simulink model "HvCoorn"  (R2022b)
settings: configuration reference "Icar05FusaMdlCfg" (kept outside this file)
undefined symbols (not defined in the file): BMSActSt_ACChrg, BMSActSt_DCChrg, BMSActSt_disconnect, BMSActSt_offline, BMSActSt_online, BMSActSt_undefined, BMSMainNegRlySt_Clsd_SC, BMSMainNegRlySt_Open_SC, BMSMainNegRlySt_StuckInClsd_SC, BMSMainNegRlySt_StuckInOpen_SC, BMSMainPosRlySt_Clsd_SC, BMSMainPosRlySt_Open_SC, BMSMainPosRlySt_StuckInClsd_SC, BMSPrecRlySt_StuckInOpen_SC, BMSReqSt_ACChrg, BMSReqSt_DCChrg, BMSReqSt_emergencyOffline, BMSReqSt_offline, BMSReqSt_online, Chrg_stCycleBookMod_SC, Chrg_stSingleBookMod_SC, CmpgMod_stInactv_SC, DCDCActSt_buck, DCDCActSt_connected, DCDCActSt_disconnected, DCDCReqSt_buck, DCDCReqSt_standby, EngStrtStop_RefuModDft_SC, EPBActSt_Appld_SC, GearLvr_stDrvGearD_SC, GearLvr_stDrvGearN_SC, GearLvr_stDrvGearP_SC, GearLvr_stDrvGearR_SC, hpp_bACChargeLinkIni_C, hpp_bACChargeLinkOKIni_C, hpp_bAcChgEnaIni_C, hpp_bAcChgPauseIni_C, hpp_bAcLinkTempErrIni_C, hpp_bBattWarmReqIni_C, hpp_bHvilHwErrIni_C, hpp_bHvilStOkIni_C, hpp_bHvRelayClsActIni_C, hpp_bHvRelayOpnActIni_C, hpp_bHvRelayStuckIni_C, hpp_bParked4ChDchgIni_C, hpp_bRemLvBatMntnReqIni_C, hpp_bStartUpReqIni_C, hpp_stHvilCanIni_C, hpp_stWarmTimeCfgRespIni_C, HvCoorn_bAuthEnaSwt_C, HvCoorn_bAuthFailSpdLimOvrd_C, HvCoorn_bAuthFailSpdLimOvrdVal_C, HvCoorn_bAuthStrt_C, HvCoorn_bBMSUnexpdDcnctFailEna_C, HvCoorn_bBuck2RdyBypDCDCEna_C, HvCoorn_bDCChrgFctCfg_C, HvCoorn_bDcChrgWkupEnaChrgLink_C, HvCoorn_bDCDcnct4ACEna_C, HvCoorn_bDCNotBuck2ShtdwnEna_C, HvCoorn_bDrvrLevNotRdyEna_C ... (+295)
libraries: ITKLib x213, simulink x61
(part 5 of 12)

== system HvCoorn/HvCoorn/HVP_HighVoltagePowerOnOffProcedure/A04_HVReq2DCBuckCal ==
  note: Documentation
  icfm_uAct : Inport
  icdc_uHvAct : Inport  Port=2
  icfm_stMode : Inport  Port=3
  icdc_stMode : Inport  Port=4
  icobc_stOBCMode : Inport  Port=5
  HvCoorn_stHVPOld : Inport  Port=6
  icobc_stChrgrCnct : Inport  Port=7
  idi_bKeyOn : Inport  Port=8
  HvCoorn_bStartUpReq : Inport  Port=9
  HvCoorn_bHvRlyClsAct : Inport  Port=10
  icrm_uAct : Inport  Port=11
  icrm_stMode : Inport  Port=12
  icbms_stDcChrg : Inport  Port=13
  icbms_stDcChrgrCnct : Inport  Port=14
  HvCoorn_stStartUpReq : Inport  Port=15
  icisg_uAct : Inport  Port=16
  VehCfg_bFrntMotByp : Inport  Port=17
  AND : Logic  OutDataTypeStr=boolean
  Constant1 : Constant  Description=[2]  Value=OBCChrgrCnctnSt_PtlCnct_SC
      settings: AttributesFormatString=%<Description>
  Constant10 : Constant  Description=[1]  Value=OBCChrgrCnctnSt_Cnct_SC
      settings: AttributesFormatString=%<Description>
  Copyright : simulink/Model-Wide Utilities/Model Info  Frame=on  DisplayStringWithTags=|  HorizontalTextAlignment=Left  LeftAlignmentValue=0.02
      | © ITK Engineering Technology (Wu Xi) Co., Ltd. (ITKC)
      | 
      | Model Version: %<ModelVersion>
      | Date: %<LastModificationDate>
  Equal : RelationalOperator  Operator=>  OutDataTypeStr=boolean  RndMeth=Simplest  InputSameDT=off
  InlineDescription : ITKLib/Special/InlineDescription  Tag=HideFromReport  Description=高压请求跳转至DCDC Buck  ShowInLibBrowser=0  RefreshPar=0
      settings: SourceProductName=ITKC_Lib
  Logical Operator1 : Logic  Inputs=3  AllPortsSameDT=off  OutDataTypeStr=boolean
  Logical Operator{5..7,10} (4 alike) : Logic  Operator=NOT  Inputs=1  AllPortsSameDT=off  OutDataTypeStr=boolean
  Logical Operator12 : Logic  Inputs=5  AllPortsSameDT=off  OutDataTypeStr=boolean
  Logical Operator{2..3,9,13,16..18} (7 alike) : Logic  Operator=OR  AllPortsSameDT=off  OutDataTypeStr=boolean
  Logical Operator{4,8,15,20} (4 alike) : Logic  AllPortsSameDT=off  OutDataTypeStr=boolean
  Min : MinMax  Function=max  Inputs=4  InputSameDT=on  SaturateOnIntegerOverflow=on
  OR : Logic  Operator=OR  OutDataTypeStr=boolean
  OR1 : Logic  Operator=OR  OutDataTypeStr=boolean
  RSLatch : ITKLib/Memory/RSLatch
      settings: SourceProductName=ITKC_Lib
  Relational Operator1 : RelationalOperator  OutDataTypeStr=boolean  InputSameDT=off
  Relational Operator{2,8,10..11,13..14} (6 alike) : RelationalOperator  Operator===  OutDataTypeStr=boolean  InputSameDT=off
  Relational Operator{3,6..7,9,12,15} (6 alike) : RelationalOperator  Operator===  OutDataTypeStr=boolean
  Switch1 : Switch  Criteria=u2 ~= 0  SaturateOnIntegerOverflow=off  InputSameDT=off
  Switch2 : Switch  Criteria=u2 ~= 0  SaturateOnIntegerOverflow=off  InputSameDT=off
  Switch3 : Switch  Criteria=u2 ~= 0  SaturateOnIntegerOverflow=off  InputSameDT=off
  TRUE : Constant  Description=TRUE  OutDataTypeStr=boolean
      settings: AttributesFormatString=%<Description>
  TRUE1 : Constant  Description=TRUE  OutDataTypeStr=boolean
      settings: AttributesFormatString=%<Description>
  TRUE2 : Constant  Description=TRUE  OutDataTypeStr=boolean
      settings: AttributesFormatString=%<Description>
  TaskTime_s2 : Constant  Value=TaskTime_10ms
      settings: AttributesFormatString=[0.01]
  TurnOnDelayVari : ITKLib/TimeCounter/TurnOnDelayVari
      settings: AttributesFormatString=TurnOnDelay  SourceProductName=ITKC_Lib
  Unit Delay : UnitDelay  SampleTime=-1  HasFrameUpgradeWarning=on
      settings: AttributesFormatString=<initial=%<x0>>
  Unit detailed design : simulink/Model-Wide Utilities/DocBlock  Tag=HideFromReport  DocumentType=Text
      content=|
      | SMiVCU-3286 - 高压连接OK标志位
      | 若以下条件同时满足，则激活[高压连接OK标志位]:
      | 1.[高压继电器闭合标志位]；
      | 2.<后电机电压>、<前电机电压>（两驱时屏蔽）和<DCDC输入电压>均大于一定值（HvCoorn_uThd4PreChrg_C，初始值220V）；
      | 3.<后电机状态>、<前电机状态>（两驱时屏蔽）均为0x3：Ready；
      | 4.<DCDC状态>为0x2：Connected；
      | 5.<OBC充电连接状态>为0x2：Connected、0x3：V2VConnected、0x4：V2LConnected且<整车电源模式>为0x0：Key Off时<OBC状态>为0x2：Connected；
      | 6.<DC充电连接状态>为0x1：WakeupInactive、0x2：WakeupActive且<整车电源模式>为0x0：Key Off时<DC充电状态>为0x0：Inactive、0x1：Active
      |
      | SMiVCU-3285 - 上高压失败标志位
      | [高压连接OK标志位]为0，且上一时刻<高压系统状态>为0x12，TurnOnDelay 一定时间（HvCoorn_tiHvOnFailSet_C，初始值2s）后激活并锁存[上高压失败标志位]，待[上高压需求标志位]出现上升沿后Reset。
      |
      | SMiVCU-3287 - 高压请求跳转至DCDCBuck标志位
      | 以下条件同时满足，则激活[高压请求跳转至DCDCBuck标志位]：
      | 1.[上高压需求标志位]为1；
      | 2.[高压连接OK标志位]为1；
      | 3.[高压失败标志位]为0；
      |
      | SMiVCU-3280 - 高压请求跳转至下电标志位
      | 若[上高压失败标志位]为1或[上高压需求标志位]为0，则激活[高压请求跳转至下电标志位]。
  icdc_connected : Constant  Description=[2]  Value=DCDCActSt_connected
      settings: AttributesFormatString=[2]
  icm_ready : Constant  Description=[3]  Value=MCUActSt_ready
      settings: AttributesFormatString=[3]
  icm_ready1 : Constant  Description=[3]  Value=MCUActSt_ready
      settings: AttributesFormatString=[3]
  icobc_connected : Constant  Description=[2]  Value=OBCActSt_connected
      settings: AttributesFormatString=[2]
  icobc_connected1 : Constant  Description=[2]  Value=OBCActSt_charging
      settings: AttributesFormatString=[3]
  sup_bHvCompReadyEnaMan_C : Constant  Description=[0]  Value=HvCoorn_bHvCptRdyEnaMan_C
      settings: AttributesFormatString=%<Description>
  sup_tiHvOnFailSet_C : Constant  Description=[5]  Value=HvCoorn_tiHvOnFailSet_C
      settings: AttributesFormatString=%<Description>
  sup_uThres_C : Constant  Description=[220]  Value=HvCoorn_uThd4PreChrg_C
      settings: AttributesFormatString=%<Description>
  sup_vLowBatVoltLim_C1 : Constant  Description=[1]  Value=HvCoorn_bHvOnDCDCByp_C
      settings: AttributesFormatString=%<Description>
  sup_vLowBatVoltLim_C2 : Constant  Description=[1]  Value=HvCoorn_bHvOnFailMCUModByp_C
      settings: AttributesFormatString=%<Description>
  sup_vLowBatVoltLim_C4 : Constant  Description=[1]  Value=HvCoorn_bHvOnFailChrgStatByp_C
      settings: AttributesFormatString=%<Description>
  uint2 : Constant  Description=HvContactorRequest  Value=12  OutDataTypeStr=uint8
      settings: AttributesFormatString=|
      | %<OutDataTypeStr>
      | %<Description>
  uint3 : Constant  Description=NoActive  Value=0  OutDataTypeStr=uint8
      settings: AttributesFormatString=|
      | %<OutDataTypeStr>
      | %<Description>
  uint4 : Constant  Description=Active  OutDataTypeStr=uint8
      settings: AttributesFormatString=|
      | %<OutDataTypeStr>
      | %<Description>
  uint5 : Constant  Description=DCPlug_WakeupInactive  OutDataTypeStr=uint8
      settings: AttributesFormatString=|
      | %<OutDataTypeStr>
      | %<Description>
  uint6 : Constant  Description=DCPlug_WakeupActive  Value=2  OutDataTypeStr=uint8
      settings: AttributesFormatString=|
      | %<OutDataTypeStr>
      | %<Description>
  HvCoorn_bHVReq2DCBuck : Outport  VectorParamsAs1DForOutWhenUnconnected=off
  HvCoorn_bHVReq2ShutDown : Outport  Port=2  VectorParamsAs1DForOutWhenUnconnected=off
  HvCoorn_bHvOnFail : Outport  Port=3  VectorParamsAs1DForOutWhenUnconnected=off
  HvCoorn_bHvOnFailRst : Outport  Port=4  VectorParamsAs1DForOutWhenUnconnected=off
  HvCoorn_bObcChrgrCnct : Outport  Port=5  VectorParamsAs1DForOutWhenUnconnected=off
  wires:
  icfm_stMode/1 -> Relational Operator2/1
  icm_ready/1 -> Relational Operator2/2
  Logical Operator2/1 -> Logical Operator5/1, Logical Operator1/2
  sup_bHvCompReadyEnaMan_C/1 -> Logical Operator2/2
  icdc_stMode/1 -> Relational Operator6/1
  icdc_connected/1 -> Relational Operator6/2
  icobc_stOBCMode/1 -> Relational Operator7/1, Relational Operator3/1
  icobc_connected/1 -> Relational Operator7/2
  Logical Operator17/1 -> Logical Operator12/4
  Switch3/1 -> AND/1
  Logical Operator12/1 -> Logical Operator2/1  "HvCoorn_bHvLinkOk"
  uint2/1 -> Relational Operator8/2
  HvCoorn_stHVPOld/1 -> Relational Operator8/1
  Logical Operator5/1 -> Logical Operator4/1
  Relational Operator8/1 -> Logical Operator4/2
  Logical Operator4/1 -> TurnOnDelayVari/1
  TurnOnDelayVari/1 -> RSLatch/1
  sup_tiHvOnFailSet_C/1 -> TurnOnDelayVari/3
  HvCoorn_bStartUpReq/1 -> Logical Operator1/1, [HvCoorn_bStartUpReq]
  idi_bKeyOn/1 -> Logical Operator7/1
  Logical Operator7/1 -> Logical Operator15/1, Logical Operator8/2
  Logical Operator8/1 -> Switch3/2
  Logical Operator18/1 -> Switch3/1
  TRUE/1 -> Switch3/3
  HvCoorn_bHvRlyClsAct/1 -> Logical Operator12/1
  Logical Operator1/1 -> HvCoorn_bHVReq2DCBuck/1  "HvCoorn_bHVReq2DCBuck"
  Logical Operator6/1 -> Logical Operator1/3
  Logical Operator9/1 -> HvCoorn_bHVReq2ShutDown/1  "HvCoorn_bHVReq2ShutDown"
  Logical Operator10/1 -> Logical Operator9/1
  RSLatch/1 -> HvCoorn_bHvOnFail/1, Logical Operator6/1, Logical Operator9/2
  sup_uThres_C/1 -> Relational Operator1/2
  icfm_uAct/1 -> Min/1
  Logical Operator13/1 -> Logical Operator12/3
  Relational Operator1/1 -> Logical Operator12/2
  [HvCoorn_bStartUpReq] -> Logical Operator10/1
  TaskTime_s2/1 -> TurnOnDelayVari/2
  icrm_uAct/1 -> Min/2
  Min/1 -> Relational Operator1/1
  icrm_stMode/1 -> Relational Operator12/1
  Relational Operator12/1 -> Logical Operator20/2
  icm_ready1/1 -> Relational Operator12/2
  uint5/1 -> Relational Operator11/2
  uint6/1 -> Relational Operator10/2
  icbms_stDcChrgrCnct/1 -> Relational Operator11/1, Relational Operator10/1
  Relational Operator11/1 -> Logical Operator3/1
  Relational Operator10/1 -> Logical Operator3/2
  Logical Operator3/1 -> Logical Operator15/2
  Logical Operator15/1 -> Switch2/2
  Switch2/1 -> AND/2
  TRUE1/1 -> Switch2/3
  uint3/1 -> Relational Operator13/2
  icbms_stDcChrg/1 -> Relational Operator13/1, Relational Operator14/1
  Relational Operator13/1 -> Logical Operator16/1
  Logical Operator16/1 -> Switch2/1
  uint4/1 -> Relational Operator14/2
  Relational Operator14/1 -> Logical Operator16/2
  Equal/1 -> RSLatch/2, HvCoorn_bHvOnFailRst/1
  Relational Operator2/1 -> Switch1/3
  Relational Operator6/1 -> Logical Operator17/1
  sup_vLowBatVoltLim_C1/1 -> Logical Operator17/2
  Relational Operator7/1 -> Logical Operator18/1
  Relational Operator3/1 -> Logical Operator18/2
  icobc_connected1/1 -> Relational Operator3/2
  HvCoorn_stStartUpReq/1 -> Equal/1, Unit Delay/1
  Unit Delay/1 -> Equal/2
  sup_vLowBatVoltLim_C2/1 -> Logical Operator13/2
  AND/1 -> OR/1
  sup_vLowBatVoltLim_C4/1 -> OR/2
  OR/1 -> Logical Operator12/5
  Constant1/1 -> Relational Operator9/2
  Relational Operator9/1 -> OR1/2
  Relational Operator15/1 -> OR1/1
  icobc_stChrgrCnct/1 -> Relational Operator15/1, Relational Operator9/1
  Constant10/1 -> Relational Operator15/2
  OR1/1 -> [HvCoorn_bObcChrgrCnct], HvCoorn_bObcChrgrCnct/1
  [HvCoorn_bObcChrgrCnct] -> Logical Operator8/1
  Logical Operator20/1 -> Logical Operator13/1
  Switch1/1 -> Logical Operator20/1
  VehCfg_bFrntMotByp/1 -> Switch1/2
  TRUE2/1 -> Switch1/1
  icdc_uHvAct/1 -> Min/3
  icisg_uAct/1 -> Min/4

== system HvCoorn/HvCoorn/HVP_HighVoltagePowerOnOffProcedure/A05_DCDCBuck2ReadyCal ==
  note: Documentation
  HvCoorn_tiHVPStTimer : Inport
  HvCoorn_bStartUpReq : Inport  Port=2
  icdc_stMode : Inport  Port=3
  HvCoorn_stHVPOld : Inport  Port=4
  AND : Logic  Inputs=4  OutDataTypeStr=boolean
  Copyright : simulink/Model-Wide Utilities/Model Info  Frame=on  DisplayStringWithTags=|  HorizontalTextAlignment=Left  LeftAlignmentValue=0.02
      | © ITK Engineering Technology (Wu Xi) Co., Ltd. (ITKC)
      | 
      | Model Version: %<ModelVersion>
      | Date: %<LastModificationDate>
  InlineDescription : ITKLib/Special/InlineDescription  Tag=HideFromReport  Description=DCDC Buck跳转至高压Ready  ShowInLibBrowser=0  RefreshPar=0
      settings: SourceProductName=ITKC_Lib
  Logical Operator : Logic  Inputs=3  AllPortsSameDT=off  OutDataTypeStr=boolean
  Logical Operator1 : Logic  Operator=OR  AllPortsSameDT=off  OutDataTypeStr=boolean
  Logical Operator2 : Logic  Operator=OR  AllPortsSameDT=off  OutDataTypeStr=boolean
  NOT : Logic  Operator=NOT  AllPortsSameDT=off  OutDataTypeStr=boolean
  NOT1 : Logic  Operator=NOT  AllPortsSameDT=off  OutDataTypeStr=boolean
  Relational Operator : RelationalOperator  Operator=>  OutDataTypeStr=boolean  InputSameDT=off
  Relational Operator1 : RelationalOperator  Operator===  OutDataTypeStr=boolean  InputSameDT=off
  Relational Operator2 : RelationalOperator  Operator=>  OutDataTypeStr=boolean  InputSameDT=off
  Relational Operator3 : RelationalOperator  Operator===  OutDataTypeStr=boolean  InputSameDT=off
  Unit detailed design : simulink/Model-Wide Utilities/DocBlock  Tag=HideFromReport  DocumentType=Text
      content=|
      | SMiVCU-3290 - DCDC Buck跳转至高压Ready标志位
      | 以下条件同时满足，则激活[DCDC Buck跳转至高压Ready标志位]：
      | 1.[上高压需求标志位]为1；
      | 2.[状态持续时间]大于一定值（HvCoorn_tiWait4Comm_C，初始值0.02s）；
      | 3.<DCDC状态>为0x3：Buck。
      |
      | SMiVCU-3291 - DCDC Buck跳转至下电标志位
      | 以下条件同时满足，或[上高压需求标志位]为0则激活[DCDC Buck跳转至下电标志位]：
      | 1.<DCDC状态>不为0x3：Buck；
      | 2.上一时刻<高压系统状态>为0x17：DCDC Buck Req；
      | 3.[状态持续时间]大于一定值（HvCoorn_tiMaxWait4DCBuck_C，初始值2s）。
  icdc_buckDcdc : Constant  Description=[3]  Value=DCDCActSt_buck
      settings: AttributesFormatString=[3]
  sup_bDCDCBuckEnaMan_C1 : Constant  Description=[0]  Value=HvCoorn_bDCNotBuck2ShtdwnEna_C
      settings: AttributesFormatString=%<Description>
  sup_tiWait4Comm_C : Constant  Description=[0.02]  Value=HvCoorn_tiWait4Comm_C
      settings: AttributesFormatString=%<Description>
  sup_tiWait4Comm_C1 : Constant  Description=[2]  Value=HvCoorn_tiMaxWait4DCBuck_C
      settings: AttributesFormatString=%<Description>
  sup_vLowBatVoltLim_C3 : Constant  Description=[1]  Value=HvCoorn_bBuck2RdyBypDCDCEna_C
      settings: AttributesFormatString=%<Description>
  uint8 : Constant  Description=DCDCBuckReq  Value=17  OutDataTypeStr=uint8
      settings: AttributesFormatString=|
      | %<OutDataTypeStr>
      | %<Description>
  HvCoorn_bDCBuck2Rdy : Outport  VectorParamsAs1DForOutWhenUnconnected=off
  HvCoorn_bDCBuck2Shtdwn : Outport  Port=2  VectorParamsAs1DForOutWhenUnconnected=off
  wires:
  sup_tiWait4Comm_C/1 -> Relational Operator/2
  Relational Operator/1 -> Logical Operator/2
  Logical Operator/1 -> HvCoorn_bDCBuck2Rdy/1  "HvCoorn_bDCBuck2Rdy"
  HvCoorn_tiHVPStTimer/1 -> [HvCoorn_tiHVPStTimer], Relational Operator/1
  Logical Operator1/1 -> Logical Operator/3
  sup_vLowBatVoltLim_C3/1 -> Logical Operator1/2
  icdc_stMode/1 -> Relational Operator3/1
  icdc_buckDcdc/1 -> Relational Operator3/2
  Relational Operator3/1 -> NOT1/1, Logical Operator1/1
  NOT/1 -> Logical Operator2/2
  HvCoorn_stHVPOld/1 -> Relational Operator1/1
  uint8/1 -> Relational Operator1/2
  AND/1 -> Logical Operator2/1
  HvCoorn_bStartUpReq/1 -> [HvCoorn_bStartUpReq], Logical Operator/1
  [HvCoorn_bStartUpReq] -> NOT/1
  sup_tiWait4Comm_C1/1 -> Relational Operator2/2
  [HvCoorn_tiHVPStTimer] -> Relational Operator2/1
  Relational Operator2/1 -> AND/4
  NOT1/1 -> AND/2
  Relational Operator1/1 -> AND/3
  sup_bDCDCBuckEnaMan_C1/1 -> AND/1
  Logical Operator2/1 -> HvCoorn_bDCBuck2Shtdwn/1  "HvCoorn_bDCBuck2Shtdwn"

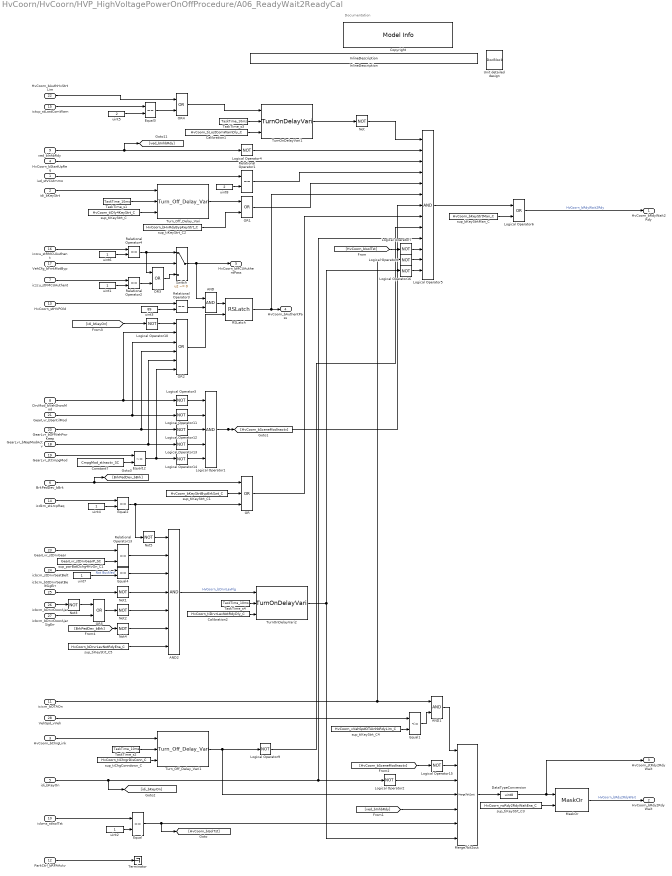
== system HvCoorn/HvCoorn/HVP_HighVoltagePowerOnOffProcedure/A06_ReadyWait2ReadyCal ==
  note: Documentation
  iud_stVCUImmo : Inport
  idi_bKeyStrt : Inport  Port=2
  HvCoorn_bChrgLink : Inport  Port=3
  HvCoorn_bStartUpReq : Inport  Port=4
  idi_bKeyOn : Inport  Port=5
  BrkPedDev_bBrk : Inport  Port=6
  iczcu_stFMCUAuthent : Inport  Port=7
  DrvMod_bVehShowMod : Inport  Port=8
  ved_bInhbRdy : Inport  Port=9
  icbms_stIsolTst : Inport  Port=10
  icicm_bOTAOn : Inport  Port=11
  ParkCtrl_bRPAActv : Inport  Port=12
  HvCoorn_stHVPOld : Inport  Port=13
  icdkm_stLrcpReq : Inport  Port=14
  ictcp_stLostComWarn : Inport  Port=15
  iczcu_stRMCUAuthent : Inport  Port=16
  VehCfg_bFrntMotByp : Inport  Port=17
  GearLvr_bNapModActv : Inport  Port=18
  GearLvr_stCmpgMod : Inport  Port=19
  GearLvr_bOffVehPwrKeep : Inport  Port=20
  GearLvr_bSentilMod : Inport  Port=21
  HvCoorn_bAuthHvStrtLim : Inport  Port=22
  GearLvr_stDrvGear : Inport  Port=23
  icbcm_stDrvrSeatBelt : Inport  Port=24
  icbcm_bStDrvrSeatBeltSigErr : Inport  Port=25
  icbcm_bDrvrDoorAjar : Inport  Port=26
  icbcm_bDrvrDoorAjarSigErr : Inport  Port=27
  VehSpd_vVeh : Inport  Port=28
  AND : Logic  OutDataTypeStr=boolean
  AND1 : Logic  OutDataTypeStr=boolean
  AND2 : Logic  Inputs=7  OutDataTypeStr=boolean
  Calibration1 : Constant  Description=[0.03]  Value=HvCoorn_tiLostComWarnDly_C  SampleTime=-1
      settings: AttributesFormatString=%<Description>
  Calibration2 : Constant  Description=[30]  Value=HvCoorn_tiDrvrLevNotRdyDly_C  SampleTime=-1
      settings: AttributesFormatString=%<Description>
  Constant7 : Constant  Description=[0]  Value=CmpgMod_stInactv_SC  SampleTime=-1
      settings: AttributesFormatString=%<Description>
  Copyright : simulink/Model-Wide Utilities/Model Info  Frame=on  DisplayStringWithTags=|  HorizontalTextAlignment=Left  LeftAlignmentValue=0.02
      | © ITK Engineering Technology (Wu Xi) Co., Ltd. (ITKC)
      | 
      | Model Version: %<ModelVersion>
      | Date: %<LastModificationDate>
  DataTypeConversion : DataTypeConversion  OutDataTypeStr=uint8  RndMeth=Nearest  SaturateOnIntegerOverflow=off
  Equal{,2..4} (4 alike) : RelationalOperator  Operator===  OutDataTypeStr=boolean  RndMeth=Simplest  InputSameDT=off
  Equal1 : RelationalOperator  Operator=<=  OutDataTypeStr=boolean  RndMeth=Simplest  InputSameDT=off
  Equal12 : RelationalOperator  Operator=~=  OutDataTypeStr=boolean
  InlineDescription : ITKLib/Special/InlineDescription  Tag=HideFromReport  Description=Ready Wait跳转至Ready  ShowInLibBrowser=0  RefreshPar=0
      settings: SourceProductName=ITKC_Lib
  Logical Operator1 : Logic  Inputs=5  AllPortsSameDT=off  OutDataTypeStr=boolean
  Logical Operator{2..4,7..16} (13 alike) : Logic  Operator=NOT  Inputs=1  AllPortsSameDT=off  OutDataTypeStr=boolean
  Logical Operator5 : Logic  Inputs=13  AllPortsSameDT=off  OutDataTypeStr=boolean
  Logical Operator6 : Logic  Operator=OR  AllPortsSameDT=off  OutDataTypeStr=boolean
  MaskOr : ITKLib/BitOperation/MaskOr
      settings: SourceProductName=ITKC_Lib
  Merge7bit2out : ITKLib/BitOperation/Merge7bit2out
      settings: SourceProductName=ITKC_Lib
  Not{,1..5} (6 alike) : Logic  Operator=NOT  AllPortsSameDT=off  OutDataTypeStr=boolean
  OR : Logic  Operator=OR  Inputs=3  OutDataTypeStr=boolean
  OR{1,3..5} (4 alike) : Logic  Operator=OR  OutDataTypeStr=boolean
  OR2 : Logic  Operator=OR  Inputs=6  OutDataTypeStr=boolean
  RSLatch : ITKLib/Memory/RSLatch
      settings: SourceProductName=ITKC_Lib
  Relational Operator{1..4,13} (5 alike) : RelationalOperator  Operator===  OutDataTypeStr=boolean  InputSameDT=off
  Switch : Switch  Criteria=u2 ~= 0  SaturateOnIntegerOverflow=off  InputSameDT=off
      settings: AttributesFormatString=Criteria : %<Criteria>
  TaskTime_s{1..4} (4 alike) : Constant  Value=TaskTime_10ms
      settings: AttributesFormatString=[0.01]
  Terminator : Terminator
  TurnOnDelayVari1 : ITKLib/TimeCounter/TurnOnDelayVari
      settings: AttributesFormatString=TurnOnDelay  SourceProductName=ITKC_Lib
  TurnOnDelayVari2 : ITKLib/TimeCounter/TurnOnDelayVari
      settings: AttributesFormatString=TurnOnDelay  SourceProductName=ITKC_Lib
  Turn_Off_Delay_Vari : ITKLib/TimeCounter/Turn_Off_Delay_Vari
      settings: AttributesFormatString=TurnOffDelay  SourceProductName=ITKC_Lib
  Turn_Off_Delay_Vari1 : ITKLib/TimeCounter/Turn_Off_Delay_Vari
      settings: AttributesFormatString=TurnOffDelay  SourceProductName=ITKC_Lib
  Unit detailed design : simulink/Model-Wide Utilities/DocBlock  Tag=HideFromReport  DocumentType=Text
      content=|
      | SMiVCU-3293 - Ready Wait跳转至Ready标志位
      | 同时满足以下条件，则激活[Ready Wait跳转至Ready标志位]：
      | 1.[上高压需求标志位]为1；
      | 2.[制动状态]为0x1：Press；
      | 3.[充电枪连接标志位]TurnOffDelay一定时间（HvCoorn_tiChrgrDisConn_C，初始值0.5s）为0；
      |
      | SMiVCU-3294 - Ready跳转至Ready Wait标志位
      | <整车电源模式>为0x0：Off或[充电枪连接标志位]TurnOffDelay一定时间（HvCoorn_tiChrgrDisConn_C，初始值0.5s）为1，则激活[Ready跳转至Ready Wait标志位]
  sup_bKeyStrtMan_C : Constant  Description=[0]  Value=HvCoorn_bKeyStrtMan_C
      settings: AttributesFormatString=%<Description>
  sup_pwrBatDchg4HvOn_C1 : Constant  Description=[6]  Value=GearLvr_stDrvGearP_SC
      settings: AttributesFormatString=%<Description>
  sup_tiChgConndown_C : Constant  Description=[0.5]  Value=HvCoorn_tiChrgrDisConn_C
      settings: AttributesFormatString=%<Description>
  sup_tiKeyStrt_C : Constant  Description=[2]  Value=HvCoorn_tiDly4KeyStrt_C
      settings: AttributesFormatString=%<Description>
  sup_tiKeyStrt_C1 : Constant  Description=[0]  Value=HvCoorn_bKeyStrtBypBrkSwt_C
      settings: AttributesFormatString=%<Description>
  sup_tiKeyStrt_C2 : Constant  Description=[1]  Value=HvCoorn_bHvRdyBypKeyStrt_C
      settings: AttributesFormatString=%<Description>
  sup_tiKeyStrt_C3 : Constant  Description=[63]  Value=HvCoorn_noRdy2RdyWaitEna_C
      settings: AttributesFormatString=%<Description>
  sup_tiKeyStrt_C4 : Constant  Description=[3]  Value=HvCoorn_vVehSpdOTAInhbRdyLim_C
      settings: AttributesFormatString=%<Description>
  sup_tiKeyStrt_C5 : Constant  Description=[1]  Value=HvCoorn_bDrvrLevNotRdyEna_C
      settings: AttributesFormatString=%<Description>
  uint1 : Constant  Description=Authentication successed  OutDataTypeStr=uint8
      settings: AttributesFormatString=|
      | %<OutDataTypeStr>
      | %<Description>
  uint2 : Constant  Description=IsolationTesting request  OutDataTypeStr=uint8
      settings: AttributesFormatString=|
      | %<OutDataTypeStr>
      | %<Description>
  uint3 : Constant  Description=Authentication successed  Value=89  OutDataTypeStr=uint8
      settings: AttributesFormatString=|
      | %<OutDataTypeStr>
      | %<Description>
  uint4 : Constant  Description=Authentication successed  OutDataTypeStr=uint8
      settings: AttributesFormatString=|
      | %<OutDataTypeStr>
      | %<Description>
  uint5 : Constant  Value=2  OutDataTypeStr=uint8  SampleTime=-1
      settings: AttributesFormatString=%<OutDataTypeStr>
  uint6 : Constant  Description=Authentication successed  OutDataTypeStr=uint8
      settings: AttributesFormatString=|
      | %<OutDataTypeStr>
      | %<Description>
  uint7 : Constant  OutDataTypeStr=uint8  SampleTime=-1
      settings: AttributesFormatString=%<OutDataTypeStr>
  uint8 : Constant  Description=Released  Value=2  OutDataTypeStr=uint8
      settings: AttributesFormatString=|
      | %<OutDataTypeStr>
      | %<Description>
  HvCoorn_bRdyWait2Rdy : Outport  VectorParamsAs1DForOutWhenUnconnected=off
  HvCoorn_bRdy2RdyWait : Outport  Port=2  VectorParamsAs1DForOutWhenUnconnected=off
  HvCoorn_stRdy2RdyWait : Outport  Port=3  VectorParamsAs1DForOutWhenUnconnected=off
  HvCoorn_bAuthentPass : Outport  Port=4  VectorParamsAs1DForOutWhenUnconnected=off
  HvCoorn_bMCUAuthentPass : Outport  Port=5  VectorParamsAs1DForOutWhenUnconnected=off
  wires:
  sup_tiKeyStrt_C/1 -> Turn_Off_Delay_Vari/3
  Turn_Off_Delay_Vari/1 -> OR1/1
  Logical Operator5/1 -> Logical Operator6/1
  Logical Operator9/1 -> Logical Operator5/9
  sup_tiChgConndown_C/1 -> Turn_Off_Delay_Vari1/3
  idi_bKeyStrt/1 -> Turn_Off_Delay_Vari/1
  HvCoorn_bStartUpReq/1 -> Logical Operator5/3
  HvCoorn_bChrgLink/1 -> Turn_Off_Delay_Vari1/1
  MaskOr/1 -> HvCoorn_bRdy2RdyWait/1  "HvCoorn_bRdy2RdyWait"
  Logical Operator6/1 -> HvCoorn_bRdyWait2Rdy/1  "HvCoorn_bRdyWait2Rdy"
  sup_bKeyStrtMan_C/1 -> Logical Operator6/2
  Turn_Off_Delay_Vari1/1 -> Merge7bit2out/4, Logical Operator9/1
  Logical Operator2/1 -> Merge7bit2out/3
  iud_stVCUImmo/1 -> Relational Operator1/1
  uint8/1 -> Relational Operator1/2
  Relational Operator1/1 -> Logical Operator5/4
  TaskTime_s1/1 -> Turn_Off_Delay_Vari/2
  TaskTime_s2/1 -> Turn_Off_Delay_Vari1/2
  BrkPedDev_bBrk/1 -> [BrkPedDev_bBrk], OR/1
  OR/1 -> Logical Operator5/8
  sup_tiKeyStrt_C1/1 -> OR/2
  OR1/1 -> Logical Operator5/5
  sup_tiKeyStrt_C2/1 -> OR1/2
  iczcu_stFMCUAuthent/1 -> Relational Operator2/1
  uint1/1 -> Relational Operator2/2
  RSLatch/1 -> Logical Operator5/6, HvCoorn_bAuthentPass/1
  idi_bKeyOn/1 -> [idi_bKeyOn], Logical Operator2/1, Logical Operator5/10
  [idi_bKeyOn] -> Logical Operator10/1
  DrvMod_bVehShowMod/1 -> Logical Operator3/1, OR2/2
  Logical Operator1/1 -> Logical Operator5/7, [HvCoorn_bSceneModInactv]
  Logical Operator4/1 -> Logical Operator5/2
  ved_bInhbRdy/1 -> [ved_bInhbRdy], Logical Operator4/1
  icbms_stIsolTst/1 -> Equal/1
  uint2/1 -> Equal/2
  Equal/1 -> Merge7bit2out/6, [HvCoorn_bIsolTst]
  [HvCoorn_bIsolTst] -> Logical Operator7/1
  Logical Operator7/1 -> Logical Operator5/11
  icicm_bOTAOn/1 -> AND1/1, Logical Operator8/1
  Logical Operator8/1 -> Logical Operator5/12
  AND/1 -> RSLatch/1
  Relational Operator3/1 -> AND/2
  HvCoorn_stHVPOld/1 -> Relational Operator3/1
  uint3/1 -> Relational Operator3/2
  [ved_bInhbRdy] -> Merge7bit2out/5
  [HvCoorn_bSceneModInactv] -> Logical Operator15/1
  Logical Operator10/1 -> OR2/1
  OR2/1 -> RSLatch/2
  Merge7bit2out/1 -> DataTypeConversion/1
  sup_tiKeyStrt_C3/1 -> MaskOr/2
  Equal1/1 -> AND1/2
  sup_tiKeyStrt_C4/1 -> Equal1/2
  VehSpd_vVeh/1 -> Equal1/1
  AND1/1 -> Merge7bit2out/1
  icdkm_stLrcpReq/1 -> Equal2/1
  uint4/1 -> Equal2/2
  Equal2/1 -> Not5/1, OR/3
  ParkCtrl_bRPAActv/1 -> Terminator/1
  TurnOnDelayVari1/1 -> Not/1
  TaskTime_s3/1 -> TurnOnDelayVari1/2
  ictcp_stLostComWarn/1 -> Equal3/1
  uint5/1 -> Equal3/2
  Calibration1/1 -> TurnOnDelayVari1/3
  Not/1 -> Logical Operator5/1
  DataTypeConversion/1 -> HvCoorn_stRdy2RdyWait/1, MaskOr/1
  uint6/1 -> Relational Operator4/2
  iczcu_stRMCUAuthent/1 -> Relational Operator4/1
  VehCfg_bFrntMotByp/1 -> Switch/2
  Switch/1 -> HvCoorn_bMCUAuthentPass/1, AND/1
  OR3/1 -> Switch/3
  Relational Operator2/1 -> OR3/2
  Relational Operator4/1 -> OR3/1, Switch/1
  Logical Operator3/1 -> Logical Operator1/1
  Logical Operator11/1 -> Logical Operator1/2
  GearLvr_bNapModActv/1 -> OR2/5, Logical Operator13/1
  GearLvr_stCmpgMod/1 -> Equal12/1
  Constant7/1 -> Equal12/2
  Equal12/1 -> OR2/6, Logical Operator14/1
  Logical Operator12/1 -> Logical Operator1/3
  GearLvr_bOffVehPwrKeep/1 -> Logical Operator12/1, OR2/4
  Logical Operator13/1 -> Logical Operator1/4
  GearLvr_bSentilMod/1 -> Logical Operator11/1, OR2/3
  Logical Operator14/1 -> Logical Operator1/5
  Logical Operator15/1 -> Merge7bit2out/2
  Equal3/1 -> OR4/2
  OR4/1 -> TurnOnDelayVari1/1
  HvCoorn_bAuthHvStrtLim/1 -> OR4/1
  GearLvr_stDrvGear/1 -> Relational Operator13/1
  sup_pwrBatDchg4HvOn_C1/1 -> Relational Operator13/2
  icbcm_stDrvrSeatBelt/1 -> Equal4/1
  uint7/1 -> Equal4/2  "Not Buckled"
  icbcm_bStDrvrSeatBeltSigErr/1 -> Not1/1
  icbcm_bDrvrDoorAjar/1 -> Not3/1
  Not3/1 -> OR5/1
  icbcm_bDrvrDoorAjarSigErr/1 -> OR5/2
  OR5/1 -> Not2/1
  TaskTime_s4/1 -> TurnOnDelayVari2/2
  Calibration2/1 -> TurnOnDelayVari2/3
  AND2/1 -> TurnOnDelayVari2/1  "HvCoorn_bDrvrLevFlg"
  TurnOnDelayVari2/1 -> Merge7bit2out/7, Logical Operator16/1
  Logical Operator16/1 -> Logical Operator5/13
  [BrkPedDev_bBrk] -> Not4/1
  Not5/1 -> AND2/1
  Relational Operator13/1 -> AND2/2
  Equal4/1 -> AND2/3
  Not1/1 -> AND2/4
  Not2/1 -> AND2/5
  Not4/1 -> AND2/6
  sup_tiKeyStrt_C5/1 -> AND2/7

== system HvCoorn/HvCoorn/HVP_HighVoltagePowerOnOffProcedure/A07_MindChange2ReadyCal ==
  note: Documentation
  HvCoorn_bStartUpReq : Inport
  icfm_stMode : Inport  Port=2
  HvCoorn_bHvRlyClsAct : Inport  Port=3
  icrm_stMode : Inport  Port=4
  icfm_uAct : Inport  Port=5
  icrm_uAct : Inport  Port=6
  icisg_uAct : Inport  Port=7
  Copyright : simulink/Model-Wide Utilities/Model Info  Frame=on  DisplayStringWithTags=|  HorizontalTextAlignment=Left  LeftAlignmentValue=0.02
      | © ITK Engineering Technology (Wu Xi) Co., Ltd. (ITKC)
      | 
      | Model Version: %<ModelVersion>
      | Date: %<LastModificationDate>
  Equal : RelationalOperator  OutDataTypeStr=boolean  RndMeth=Simplest  InputSameDT=off
  InlineDescription : ITKLib/Special/InlineDescription  Tag=HideFromReport  Description=MindChange跳转至Ready  ShowInLibBrowser=0  RefreshPar=0
      settings: SourceProductName=ITKC_Lib
  Logical Operator : Logic  Inputs=3  AllPortsSameDT=off  OutDataTypeStr=boolean
  Max : MinMax  Function=max  Inputs=3
  OR : Logic  Operator=OR  OutDataTypeStr=boolean
  Relational Operator1 : RelationalOperator  Operator===  OutDataTypeStr=boolean  InputSameDT=off
  Relational Operator2 : RelationalOperator  Operator===  OutDataTypeStr=boolean  InputSameDT=off
  Switch : Switch  Criteria=u2 ~= 0  SaturateOnIntegerOverflow=off  InputSameDT=off
      settings: AttributesFormatString=Criteria : %<Criteria>
  Unit detailed design : simulink/Model-Wide Utilities/DocBlock  Tag=HideFromReport  DocumentType=Text
      content=|
      | SMiVCU-3299 - MindChange跳转至Ready标志位
      | 以下条件同时满足，则激活[MindChange跳转至Ready标志位]：
      | 1.<前电机状态>为0x3：ready（两驱时屏蔽）；
      | 2.<后电机状态>为0x3：ready；
      | 3.[上高压需求标志位]为1；
      | 4.[高压继电器闭合标志位]为1；
  icm_ready : Constant  Description=[3]  Value=MCUActSt_ready
      settings: AttributesFormatString=[3]
  icm_ready1 : Constant  Description=[3]  Value=MCUActSt_ready
      settings: AttributesFormatString=[3]
  sup_uThres_C : Constant  Description=[220]  Value=HvCoorn_uThd4PreChrg_C
      settings: AttributesFormatString=%<Description>
  sup_uThres_C1 : Constant  Description=[1]  Value=HvCoorn_bMindChag2RdyChkMCUVolt_C
      settings: AttributesFormatString=%<Description>
  HvCoorn_bMindChag2Rdy : Outport  VectorParamsAs1DForOutWhenUnconnected=off
  wires:
  Logical Operator/1 -> HvCoorn_bMindChag2Rdy/1  "HvCoorn_bMindChag2Rdy"
  icfm_stMode/1 -> Relational Operator1/1
  icm_ready/1 -> Relational Operator1/2
  Relational Operator1/1 -> OR/1
  HvCoorn_bHvRlyClsAct/1 -> Logical Operator/3
  HvCoorn_bStartUpReq/1 -> Logical Operator/2
  icm_ready1/1 -> Relational Operator2/2
  icrm_stMode/1 -> Relational Operator2/1
  Relational Operator2/1 -> OR/2
  Switch/1 -> Logical Operator/1
  icrm_uAct/1 -> Max/2
  icfm_uAct/1 -> Max/1
  OR/1 -> Switch/3
  sup_uThres_C1/1 -> Switch/2
  Max/1 -> Equal/1
  sup_uThres_C/1 -> Equal/2
  Equal/1 -> Switch/1
  icisg_uAct/1 -> Max/3

== system HvCoorn/HvCoorn/HVP_HighVoltagePowerOnOffProcedure/A08_MindChange2ShutHVCal ==
  note: Documentation
  VehSpd_vVeh : Inport
  HvCoorn_tiHVPStTimer : Inport  Port=2
  HvCoorn_bHvRlyOpenAct : Inport  Port=3
  icfm_stMode : Inport  Port=4
  icrm_stMode : Inport  Port=5
  icdc_stMode : Inport  Port=6
  HvCoorn_bStartUpReq : Inport  Port=7
  icobc_stOBCMode : Inport  Port=8
  ved_bHvShtdwn : Inport  Port=9
  HvCoorn_stHVPOld : Inport  Port=10
  icbms_iHVBat : Inport  Port=11
  VehCfg_bFrntMotByp : Inport  Port=12
  icisg_stMod : Inport  Port=13
  1-D Lookup Table1 : Lookup_n-D  NumberOfTableDimensions=1  BreakpointsForDimension1=HvCoorn_tiWait4StdbyRdyHv_AX  BreakpointsForDimension1DataTypeStr=Inherit: Inherit from 'Breakpoint data'  Table=HvCoorn_tiWait4StdbyRdyHv_T  TableDataTypeStr=Inherit: Inherit from 'Table data'  ExtrapMethod=Clip  UseLastTableValue=on  InternalRulePriority=Speed  OutDataTypeStr=Inherit: Inherit from 'Table data'  RndMeth=Simplest
      settings: AttributesFormatString=|
      | input = %<BreakpointsForDimension1>
      | output = %<Table>
      | extrapolation-use end values: %<UseLastTableValue>
  Abs : Abs
  Abs1 : Abs
  Add : Sum  OutDataTypeStr=int8  SaturateOnIntegerOverflow=on
  Copyright : simulink/Model-Wide Utilities/Model Info  Frame=on  DisplayStringWithTags=|  HorizontalTextAlignment=Left  LeftAlignmentValue=0.02
      | © ITK Engineering Technology (Wu Xi) Co., Ltd. (ITKC)
      | 
      | Model Version: %<ModelVersion>
      | Date: %<LastModificationDate>
  EdgeRising1 : ITKLib/Memory/EdgeRising  Tag=initial value = 0
      settings: SourceProductName=ITKC_Lib
  EdgeRising2 : ITKLib/Memory/EdgeRising  Tag=initial value = 0
      settings: SourceProductName=ITKC_Lib
  InlineDescription : ITKLib/Special/InlineDescription  Tag=HideFromReport  Description=MindChange跳转至断高压  ShowInLibBrowser=0  RefreshPar=0
      settings: SourceProductName=ITKC_Lib
  Logical Operator : Logic  Inputs=3  AllPortsSameDT=off  OutDataTypeStr=boolean
  Logical Operator1 : Logic  Inputs=3  AllPortsSameDT=off  OutDataTypeStr=boolean
  Logical Operator10 : Logic  AllPortsSameDT=off  OutDataTypeStr=boolean
  Logical Operator2 : Logic  AllPortsSameDT=off  OutDataTypeStr=boolean
  Logical Operator3 : Logic  Operator=OR  Inputs=3  AllPortsSameDT=off  OutDataTypeStr=boolean
  Logical Operator4 : Logic  Operator=OR  AllPortsSameDT=off  OutDataTypeStr=boolean
  Logical Operator5 : Logic  Inputs=6  AllPortsSameDT=off  OutDataTypeStr=boolean
  Logical Operator6 : Logic  Operator=OR  AllPortsSameDT=off  OutDataTypeStr=boolean
  Logical Operator7 : Logic  AllPortsSameDT=off  OutDataTypeStr=boolean
  Logical Operator8 : Logic  Operator=NOT  Inputs=1  AllPortsSameDT=off  OutDataTypeStr=boolean
  Logical Operator9 : Logic  Operator=OR  AllPortsSameDT=off  OutDataTypeStr=boolean
  OR : Logic  Operator=OR  OutDataTypeStr=boolean
  RSLatch : ITKLib/Memory/RSLatch
      settings: SourceProductName=ITKC_Lib
  Relational Operator{1,5,8..13} (8 alike) : RelationalOperator  Operator=~=  OutDataTypeStr=boolean  InputSameDT=off
  Relational Operator15 : RelationalOperator  Operator===  OutDataTypeStr=boolean  InputSameDT=off
  Relational Operator2 : RelationalOperator  Operator=<  OutDataTypeStr=boolean  InputSameDT=off
  Relational Operator3 : RelationalOperator  Operator=>  OutDataTypeStr=boolean  InputSameDT=off
  Relational Operator4 : RelationalOperator  Operator=>  OutDataTypeStr=boolean  InputSameDT=off
  Relational Operator6 : RelationalOperator  Operator=<=  OutDataTypeStr=boolean  InputSameDT=off
  Relational Operator7 : RelationalOperator  OutDataTypeStr=boolean  InputSameDT=off
  Saturation : Saturate  UpperLimit=10  LowerLimit=0  OutDataTypeStr=int8
      settings: AttributesFormatString=<limits=%<UpperLimit>/%<LowerLimit>>
  Switch : Switch  Criteria=u2 ~= 0  SaturateOnIntegerOverflow=off  InputSameDT=off
  Switch1 : Switch  Criteria=u2 ~= 0  SaturateOnIntegerOverflow=off  InputSameDT=off
  TaskTime_s1 : Constant  Value=TaskTime_10ms
      settings: AttributesFormatString=[0.01]
  TaskTime_s3 : Constant  Value=TaskTime_10ms
      settings: AttributesFormatString=[0.01]
  TaskTime_s4 : Constant  Value=TaskTime_10ms
      settings: AttributesFormatString=[0.01]
  TurnOnDelayVari : ITKLib/TimeCounter/TurnOnDelayVari
      settings: AttributesFormatString=TurnOnDelay  SourceProductName=ITKC_Lib
  TurnOnDelayVari1 : ITKLib/TimeCounter/TurnOnDelayVari
      settings: AttributesFormatString=TurnOnDelay  SourceProductName=ITKC_Lib
  TurnOnDelayVari2 : ITKLib/TimeCounter/TurnOnDelayVari
      settings: AttributesFormatString=TurnOnDelay  SourceProductName=ITKC_Lib
  Unit Delay : UnitDelay  SampleTime=-1  HasFrameUpgradeWarning=on
      settings: AttributesFormatString=<initial=%<X0>>
  Unit Delay1 : UnitDelay  SampleTime=-1  HasFrameUpgradeWarning=on
      settings: AttributesFormatString=<initial=%<X0>>
  Unit detailed design : simulink/Model-Wide Utilities/DocBlock  Tag=HideFromReport  DocumentType=Text
      content=|
      | SMiVCU-3296 - 无高压负载标志位
      | 以下条件同时成立，则激活[无高压负载标志位]：
      | 1.<前电机状态>不为0x4：TrqCtrl（两驱时屏蔽）；
      | 2.<后电机状态>不为0x4：TrqCtrl；
      | 3.<DCDC状态>不为0x3：Buck；
      | 4.<OBC状态>不为0x3：Charging、0x4：V2L、0x5：V2V;
      | 5.<电池电流>的绝对值小于一定值（HvCoorn_iBatMax4RlyOpen_C，初始值5A）且超过一定时间（HvCoorn_tiBatCurChk4RlyOpen_C，初始值0.03s）；
      |
      | SMiVCU-3297 - MindChange跳转至断高压标志位
      | [高压继电器断开标志位]为1；或[下电请求标志位]为1且[状态持续时间]大于一定值（HvCoorn_tiTimeOutStdbyRdyHv_C，初始值5s），或以下条件同时满足，则激活[MindChange跳转至断高压标志位]:
      | 1.[状态持续时间]大于根据重新尝试上电次数查表（HvCoorn_tiWait4StdbyRdyHv_T）得到的时间；
      | 2.[无高压负载标志位]为1或[状态持续时间]大于一定值（HvCoorn_tiTimeOutStdbyRdyHv_C，初始值5s）；
      | 3.<实际车速>绝对值小于一定值（HvCoorn_v4ShutDown_C，初始值1.5kph）或不小于此值但上一时刻<高压系统状态>为95持续超过一定时间（HvCoorn_tiSpdWaitTimout_C，初始值300s）;
  Wait4MindChange : Constant  Value=95  OutDataTypeStr=uint8
  icdc_buckDcdc : Constant  Description=[3]  Value=DCDCActSt_buck  OutDataTypeStr=uint8
      settings: AttributesFormatString=[3]
  icm_trqCtrl : Constant  Description=[4]  Value=MCUActSt_trqCtrl  OutDataTypeStr=uint8
      settings: AttributesFormatString=[4]
  icm_trqCtrl1 : Constant  Description=[4]  Value=MCUActSt_trqCtrl  OutDataTypeStr=uint8
      settings: AttributesFormatString=[4]
  icobc_V2L : Constant  Description=[4]  Value=OBCActSt_V2L  OutDataTypeStr=uint8
      settings: AttributesFormatString=[4]
  icobc_V2V : Constant  Description=[5]  Value=OBCActSt_V2V  OutDataTypeStr=uint8
      settings: AttributesFormatString=[5]
  icobc_V2V1 : Constant  Description=[5]  Value=ISGModSt_SpdCtrl_SC  OutDataTypeStr=uint8
      settings: AttributesFormatString=%<Description>
  icobc_charging : Constant  Description=[3]  Value=OBCActSt_charging  OutDataTypeStr=uint8
      settings: AttributesFormatString=[3]
  icobc_charging1 : Constant  Description=[3]  Value=ISGModSt_TqCtrl_SC  OutDataTypeStr=uint8
      settings: AttributesFormatString=%<Description>
  int1 : Constant  OutDataTypeStr=int8
      settings: AttributesFormatString=%<OutDataTypeStr>
  int2 : Constant  Value=-1  OutDataTypeStr=int8
      settings: AttributesFormatString=%<OutDataTypeStr>
  int3 : Constant  Value=0  OutDataTypeStr=int8
      settings: AttributesFormatString=%<OutDataTypeStr>
  int8 : Constant  OutDataTypeStr=int8
      settings: AttributesFormatString=%<OutDataTypeStr>
  sup_iBatMax4RlyOpn_C : Constant  Description=[5]  Value=HvCoorn_iBatMax4RlyOpen_C
      settings: AttributesFormatString=%<Description>
  sup_tiBatCurChk4RlyOpn_C : Constant  Description=[0.03]  Value=HvCoorn_tiBatCurChk4RlyOpen_C
      settings: AttributesFormatString=%<Description>
  sup_tiSpdWaitTimout_C : Constant  Description=[300]  Value=HvCoorn_tiSpdWaitTimout_C
      settings: AttributesFormatString=%<Description>
  sup_tiSpdWaitTimout_C1 : Constant  Description=[0]  Value=HvCoorn_bVehSpd4HvDownByp_C
      settings: AttributesFormatString=%<Description>
  sup_tiTimeOutStandbyRdyHv_C : Constant  Description=[5]  Value=HvCoorn_tiTimeOutStdbyRdyHv_C
      settings: AttributesFormatString=%<Description>
  sup_tiWait4CountDown_C : Constant  Description=[2]  Value=HvCoorn_tiWait4CountDown_C
      settings: AttributesFormatString=%<Description>
  sup_vForShutDown_C : Constant  Description=[1.5]  Value=HvCoorn_v4ShutDown_C
      settings: AttributesFormatString=%<Description>
  HvCoorn_bMindChag2ShutHV : Outport  VectorParamsAs1DForOutWhenUnconnected=off
  HvCoorn_bVehSpd4HvDown : Outport  Port=2  VectorParamsAs1DForOutWhenUnconnected=off
  wires:
  icm_trqCtrl/1 -> Relational Operator1/2
  icfm_stMode/1 -> Relational Operator1/1
  1-D Lookup Table1/1 -> Relational Operator3/2
  HvCoorn_tiHVPStTimer/1 -> Relational Operator4/1, Relational Operator3/1
  sup_tiTimeOutStandbyRdyHv_C/1 -> Relational Operator4/2
  icdc_buckDcdc/1 -> Relational Operator5/2
  icdc_stMode/1 -> Relational Operator5/1
  VehSpd_vVeh/1 -> Abs/1
  sup_vForShutDown_C/1 -> Relational Operator6/2
  Relational Operator3/1 -> Logical Operator/1  "bCycleOk"
  Relational Operator6/1 -> Logical Operator8/1, Logical Operator6/2, Logical Operator9/1  "bSpdOk"
  HvCoorn_bHvRlyOpenAct/1 -> Logical Operator3/1
  Logical Operator2/1 -> Logical Operator3/2
  Logical Operator/1 -> Logical Operator3/3
  Logical Operator3/1 -> HvCoorn_bMindChag2ShutHV/1  "HvCoorn_bMindChag2ShutHV"
  Abs/1 -> Relational Operator6/1
  sup_iBatMax4RlyOpn_C/1 -> Relational Operator2/2
  Relational Operator2/1 -> TurnOnDelayVari1/1
  sup_tiBatCurChk4RlyOpn_C/1 -> TurnOnDelayVari1/3
  Abs1/1 -> Relational Operator2/1
  icbms_iHVBat/1 -> Abs1/1
  HvCoorn_bStartUpReq/1 -> EdgeRising1/1
  EdgeRising1/1 -> Switch/2
  int8/1 -> Switch/1
  Switch/1 -> Add/1
  Switch1/1 -> Switch/3
  RSLatch/1 -> TurnOnDelayVari/1
  sup_tiWait4CountDown_C/1 -> TurnOnDelayVari/3
  EdgeRising2/1 -> Switch1/2
  int2/1 -> Switch1/1
  int3/1 -> Switch1/3
  Add/1 -> Saturation/1
  Unit Delay/1 -> Add/2, Relational Operator7/1
  Saturation/1 -> 1-D Lookup Table1/1, Unit Delay/1
  TurnOnDelayVari/1 -> EdgeRising2/1, Unit Delay1/1
  int1/1 -> Relational Operator7/2
  Relational Operator7/1 -> RSLatch/1
  Unit Delay1/1 -> RSLatch/2
  icobc_charging/1 -> Relational Operator11/2
  icobc_stOBCMode/1 -> Relational Operator10/1, Relational Operator9/1, Relational Operator11/1
  icobc_V2V/1 -> Relational Operator10/2
  icobc_V2L/1 -> Relational Operator9/2
  Relational Operator11/1 -> Logical Operator1/1
  Relational Operator9/1 -> Logical Operator1/2
  Relational Operator10/1 -> Logical Operator1/3
  Relational Operator4/1 -> [bHvShutTimeout], Logical Operator2/2
  ved_bHvShtdwn/1 -> Logical Operator2/1
  OR/1 -> Logical Operator5/1
  Logical Operator1/1 -> Logical Operator5/4
  TurnOnDelayVari1/1 -> Logical Operator5/6
  Logical Operator5/1 -> Logical Operator4/1  "HvCoorn_bHvNoLoad"
  [bHvShutTimeout] -> Logical Operator4/2
  Logical Operator4/1 -> Logical Operator/2  "bCurrOk"
  HvCoorn_stHVPOld/1 -> Relational Operator15/1
  Wait4MindChange/1 -> Relational Operator15/2
  Logical Operator8/1 -> Logical Operator7/1
  Relational Operator15/1 -> Logical Operator7/2
  Logical Operator7/1 -> TurnOnDelayVari2/1
  sup_tiSpdWaitTimout_C/1 -> TurnOnDelayVari2/3
  TurnOnDelayVari2/1 -> Logical Operator9/2
  Logical Operator9/1 -> Logical Operator/3
  Relational Operator5/1 -> Logical Operator5/3
  TaskTime_s1/1 -> TurnOnDelayVari/2
  TaskTime_s3/1 -> TurnOnDelayVari1/2
  TaskTime_s4/1 -> TurnOnDelayVari2/2
  icm_trqCtrl1/1 -> Relational Operator8/2
  Relational Operator8/1 -> Logical Operator5/2
  icrm_stMode/1 -> Relational Operator8/1
  Relational Operator1/1 -> OR/1
  VehCfg_bFrntMotByp/1 -> OR/2
  Logical Operator6/1 -> HvCoorn_bVehSpd4HvDown/1
  sup_tiSpdWaitTimout_C1/1 -> Logical Operator6/1
  Logical Operator10/1 -> Logical Operator5/5
  Relational Operator12/1 -> Logical Operator10/1
  Relational Operator13/1 -> Logical Operator10/2
  icisg_stMod/1 -> Relational Operator12/1, Relational Operator13/1
  icobc_charging1/1 -> Relational Operator12/2
  icobc_V2V1/1 -> Relational Operator13/2

== system HvCoorn/HvCoorn/HVP_HighVoltagePowerOnOffProcedure/A09_ShutHV2ShutDisChCal ==
  note: Documentation
  HvCoorn_bHvRlyOpenAct : Inport
  icfm_nAct : Inport  Port=2
  icrm_nAct : Inport  Port=3
  icisg_nAct : Inport  Port=4
  HvCoorn_tiHVPStTimer : Inport  Port=5
  HvCoorn_stHVPOld : Inport  Port=6
  AND : Logic  OutDataTypeStr=boolean
  AND1 : Logic  OutDataTypeStr=boolean
  Abs : Abs
  Abs1 : Abs
  Abs2 : Abs
  Copyright : simulink/Model-Wide Utilities/Model Info  Frame=on  DisplayStringWithTags=|  HorizontalTextAlignment=Left  LeftAlignmentValue=0.02
      | © ITK Engineering Technology (Wu Xi) Co., Ltd. (ITKC)
      | 
      | Model Version: %<ModelVersion>
      | Date: %<LastModificationDate>
  InlineDescription : ITKLib/Special/InlineDescription  Tag=HideFromReport  Description=断高压跳转至主动放电  ShowInLibBrowser=0  RefreshPar=0
      settings: SourceProductName=ITKC_Lib
  Logical Operator2 : Logic  Operator=OR  AllPortsSameDT=off  OutDataTypeStr=boolean
  Max : MinMax  Function=max  Inputs=3  InputSameDT=on  SaturateOnIntegerOverflow=on
  Relational Operator15 : RelationalOperator  Operator===  OutDataTypeStr=boolean  InputSameDT=off
  Relational Operator4 : RelationalOperator  Operator=>  OutDataTypeStr=boolean  InputSameDT=off
  Relational Operator6 : RelationalOperator  Operator=<=  OutDataTypeStr=boolean  InputSameDT=off
  Unit detailed design : simulink/Model-Wide Utilities/DocBlock  Tag=HideFromReport  DocumentType=Text
      content=|
      | SMiVCU-3301 - 断高压跳转至主动放电标志位
      | [高压继电器断开标志位]为1，且<前后电机实际转速>的绝对值均小于一定值（HvCoorn_nMotThrd4DChrg_C，初始值60rpm），则激活[断高压跳转至主动放电标志位]；
  Wait4MindChange : Constant  Value=101  OutDataTypeStr=uint8
  sup_nMotThres4Dcha_C : Constant  Description=[60]  Value=HvCoorn_nMotThrd4DChrg_C
      settings: AttributesFormatString=%<Description>
  sup_tiTimeOutStandbyRdyHv_C : Constant  Description=[5]  Value=HvCoorn_tiTimeOutShutHv2Dchrg_C
      settings: AttributesFormatString=%<Description>
  HvCoorn_bShutHV2ShutDisCh : Outport  VectorParamsAs1DForOutWhenUnconnected=off
  wires:
  HvCoorn_bHvRlyOpenAct/1 -> AND1/1
  sup_nMotThres4Dcha_C/1 -> Relational Operator6/2
  Abs/1 -> Max/1
  icfm_nAct/1 -> Abs/1
  Relational Operator6/1 -> AND1/2
  Logical Operator2/1 -> HvCoorn_bShutHV2ShutDisCh/1  "HvCoorn_bShutHV2ShutDisCh"
  icrm_nAct/1 -> Abs1/1
  Abs1/1 -> Max/2
  Max/1 -> Relational Operator6/1
  icisg_nAct/1 -> Abs2/1
  Abs2/1 -> Max/3
  HvCoorn_tiHVPStTimer/1 -> Relational Operator4/1
  HvCoorn_stHVPOld/1 -> Relational Operator15/1
  Relational Operator15/1 -> AND/1
  Relational Operator4/1 -> AND/2
  sup_tiTimeOutStandbyRdyHv_C/1 -> Relational Operator4/2
  Wait4MindChange/1 -> Relational Operator15/2
  AND1/1 -> Logical Operator2/1
  AND/1 -> Logical Operator2/2
